simulink library "veneziane"  (R2024b)
settings: Solver=VariableStepAuto  StartTime=0.0  StopTime=10.0  RelTol=1e-3
settings Model: Creator=mainuser  LastModifiedBy=xandr

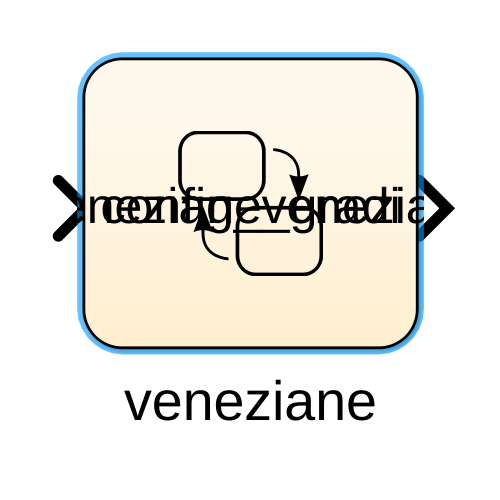
[thumbnail: Simulink's stored preview of the top-level diagram]
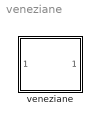
== system veneziane ==
  veneziane : Stateflow chart  TreatAsAtomicUnit=on

== stateflow chart veneziane/veneziane ==
  state Attivo
    state Attivo_ON
      en: config_mode = 1;
      config_angolo = new_angolo;
      servo_output = new_angolo
    state Attivo_OFF
      en: angolo_veneziane = config_angolo
      servo_output = config_angolo
    (default) -> Attivo_OFF [order 3] : [veneziane_button_pressed == 1]
        | {config_mode = 0;}
    (default) -> Attivo_ON [order 2] : [veneziane_button_pressed ==1]
    (default) -> Attivo_OFF [order 1]
  state Inattivo
    en:angolo_veneziane = 0;
    servo_output=0;
  (default) -> Inattivo [order 2]
  Attivo -> Inattivo : [config_veneziane_gradi == false]
  (default) -> Attivo [order 1] : [config_veneziane_gradi == true]
  data: config_veneziaone_gradi input; io_veneziane_gradi output
